simulink model "motores_cc"  (R2018a)
settings: Solver=VariableStepAuto  StartTime=0.0  StopTime=1000.0  RelTol=1e-3
settings Model: Creator=gbs  LastModifiedBy=gbs

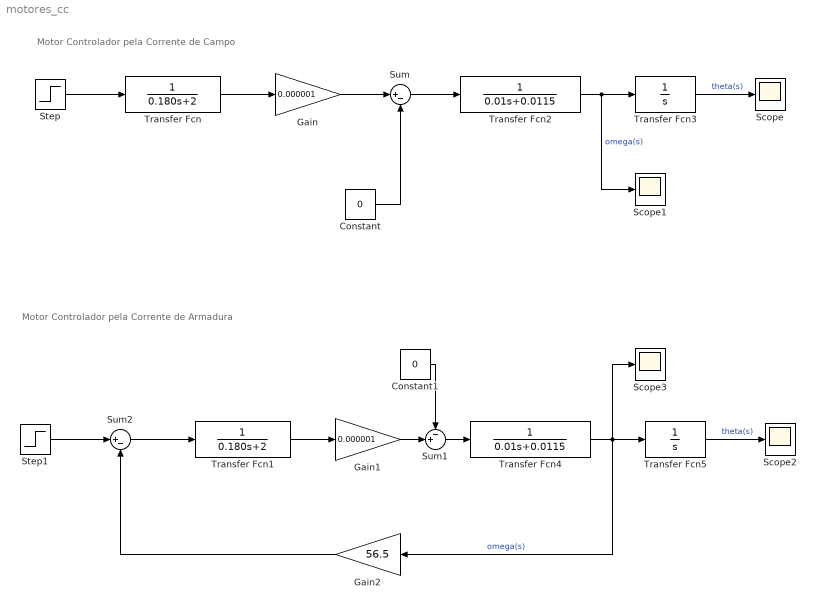
== system motores_cc ==
  note: Motor Controlador pela Corrente de Campo
  note: Motor Controlador pela Corrente de Armadura
  Constant : Constant  Value=0
  Constant1 : Constant  Value=0
  Gain : Gain  Gain=0.000001
  Gain1 : Gain  Gain=0.000001
  Gain2 : Gain  Gain=56.5
  Scope{,1..3} (4 alike) : Scope
  Step : Step  SampleTime=0
  Step1 : Step  SampleTime=0
  Sum : Sum  Inputs=|+-
  Sum1 : Sum  Inputs=-+|
  Sum2 : Sum  Inputs=|+-
  Transfer Fcn : TransferFcn  Denominator=[0.180 2]
  Transfer Fcn1 : TransferFcn  Denominator=[0.180 2]
  Transfer Fcn2 : TransferFcn  Denominator=[0.01 0.0115]
  Transfer Fcn3 : TransferFcn  Denominator=[1 0]
  Transfer Fcn4 : TransferFcn  Denominator=[0.01 0.0115]
  Transfer Fcn5 : TransferFcn  Denominator=[1 0]
  wires:
  Transfer Fcn/1 -> Gain/1
  Gain/1 -> Sum/1
  Sum/1 -> Transfer Fcn2/1
  Transfer Fcn2/1 -> Scope1/1, Transfer Fcn3/1  "omega(s)"
  Transfer Fcn3/1 -> Scope/1  "theta(s)"
  Step/1 -> Transfer Fcn/1
  Constant/1 -> Sum/2
  Transfer Fcn1/1 -> Gain1/1
  Transfer Fcn4/1 -> Scope3/1, Gain2/1, Transfer Fcn5/1  "omega(s)"
  Sum1/1 -> Transfer Fcn4/1
  Transfer Fcn5/1 -> Scope2/1  "theta(s)"
  Gain1/1 -> Sum1/2
  Constant1/1 -> Sum1/1
  Step1/1 -> Sum2/1
  Sum2/1 -> Transfer Fcn1/1
  Gain2/1 -> Sum2/2
